simulink model "Hardmon_CAN"  (R2023b)
settings: Solver=VariableStepAuto  StartTime=0.0  StopTime=10.0  RelTol=1e-3
settings Model: Creator=heyka  LastModifiedBy=heyka

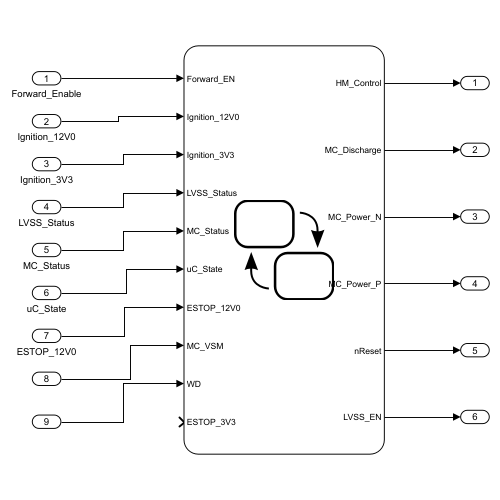
[thumbnail: Simulink's stored preview of the top-level diagram]
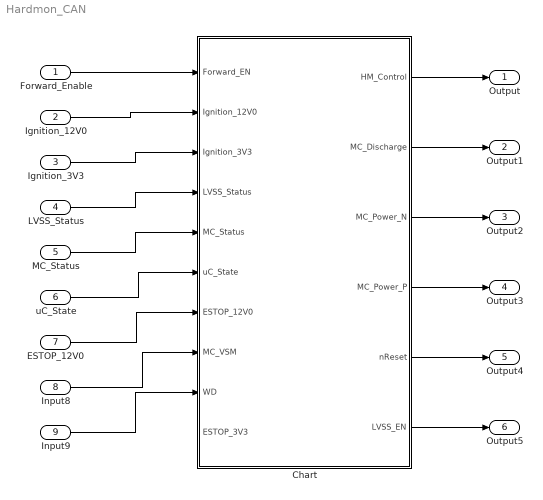
== system Hardmon_CAN ==
  Forward_Enable : Inport
  Ignition_12V0 : Inport  Port=2
  Ignition_3V3 : Inport  Port=3
  LVSS_Status : Inport  Port=4
  MC_Status : Inport  Port=5
  uC_State : Inport  Port=6
  ESTOP_12V0 : Inport  Port=7
  Input8 : Inport  Port=8
  Input9 : Inport  Port=9
  Chart : Stateflow chart  TreatAsAtomicUnit=on
  Output : Outport
  Output1 : Outport  Port=2
  Output2 : Outport  Port=3
  Output3 : Outport  Port=4
  Output4 : Outport  Port=5
  Output5 : Outport  Port=6
  wires:
  Input8/1 -> Chart/8(MC_VSM)
  uC_State/1 -> Chart/6(uC_State)
  Forward_Enable/1 -> Chart/1(Forward_EN)
  LVSS_Status/1 -> Chart/4(LVSS_Status)
  Chart/5(nReset) -> Output4/1
  Ignition_12V0/1 -> Chart/2(Ignition_12V0)
  Ignition_3V3/1 -> Chart/3(Ignition_3V3)
  ESTOP_12V0/1 -> Chart/7(ESTOP_12V0)
  MC_Status/1 -> Chart/5(MC_Status)
  Input9/1 -> Chart/9(WD)
  Chart/1(HM_Control) -> Output/1
  Chart/2(MC_Discharge) -> Output1/1
  Chart/3(MC_Power_N) -> Output2/1
  Chart/4(MC_Power_P) -> Output3/1
  Chart/6(LVSS_EN) -> Output5/1

== stateflow chart Hardmon_CAN/Chart ==
  state Normal_Operation
    state ESTOP_Checking [parallel]
      settings: executionOrder=1
      state count
        entry:
        ESTOP_Counter = ESTOP_Counter + 1;
      state ESTOP_Inactive
        entry:
        Fault = 0;
        ESTOP_Counter = 0;
        HM_Control = 0;
        LVSS_EN = 1;
      (default) -> ESTOP_Inactive
      ESTOP_Inactive -> Normal_Operation.ESTOP_Checking.count : [ESTOP_3V3 == 1]
      Normal_Operation.ESTOP_Checking.count -> ESTOP_Inactive [order 2] : [ESTOP_3V3 == 0 || uC_State == 7]
      Normal_Operation.ESTOP_Checking.count -> Normal_Operation.ESTOP_Checking.count [order 1] : after(0.5,sec)
    state Watchdog_Checking [parallel]
      settings: executionOrder=2
      state WD_Low
        entry:
        WD_Count = 0
        state Counting
          entry:
          WD_Count = WD_Count + 1
        Normal_Operation.Watchdog_Checking.WD_Low.Counting -> Normal_Operation.Watchdog_Checking.WD_Low.Counting : after(0.5, sec)
      state WD_High
        entry:
        WD_Count = 0;
        state Counting
          entry:
          WD_Count = WD_Count + 1
        Normal_Operation.Watchdog_Checking.WD_High.Counting -> Normal_Operation.Watchdog_Checking.WD_High.Counting : after(0.5, sec)
      (default) -> WD_Low
      WD_Low -> WD_High : [WD == 1]
      WD_High -> WD_Low : [WD == 0]
    state Invalid_State_Checking [parallel]
      settings: executionOrder=3
      state count
        entry:
        Invalid_State_Counter = Invalid_State_Counter + 1;
      state Invalid_State_Inactive
        entry:
        Fault = 0;
        Invalid_State_Counter = 0;
        HM_Control = 0;
        LVSS_EN = 1;
      (default) -> Normal_Operation.Invalid_State_Checking.Invalid_State_Inactive
      Normal_Operation.Invalid_State_Checking.Invalid_State_Inactive -> Normal_Operation.Invalid_State_Checking.count : [(Forward_EN ~= 1 || Ignition_3V3 ~= 1) && uC_State == 3]
      Normal_Operation.Invalid_State_Checking.count -> Normal_Operation.Invalid_State_Checking.Invalid_State_Inactive [order 2] : [~((Forward_EN ~= 1 || Ignition_3V3 ~= 1) && uC_State == 3)]
      Normal_Operation.Invalid_State_Checking.count -> Normal_Operation.Invalid_State_Checking.count [order 1] : after(0.5,sec)
    state Ignition_Level_Checking [parallel]
      settings: executionOrder=4
      state count
        entry:
        Ignition_State_Counter = Invalid_State_Counter + 1;
      state Ignition_State_Inactive
        entry:
        Fault = 0;
        Ignition_State_Counter = 0;
        HM_Control = 0;
        LVSS_EN = 1;
      (default) -> Ignition_State_Inactive
      Ignition_State_Inactive -> Normal_Operation.Ignition_Level_Checking.count : [Ignition_3V3 ~= Ignition_12V0]
      Normal_Operation.Ignition_Level_Checking.count -> Ignition_State_Inactive [order 2] : [Ignition_3V3 == Ignition_12V0]
      Normal_Operation.Ignition_Level_Checking.count -> Normal_Operation.Ignition_Level_Checking.count [order 1] : after(0.5,sec)
    state ESTOP_Level_Checking [parallel]
      settings: executionOrder=5
      state count
        entry:
        ESTOP_State_Counter = ESTOP_State_Counter + 1;
      state ESTOP_State_Inactive
        entry:
        Fault = 0;
        ESTOP_State_Counter = 0;
        HM_Control = 0;
        LVSS_EN = 1;
      (default) -> ESTOP_State_Inactive
      ESTOP_State_Inactive -> Normal_Operation.ESTOP_Level_Checking.count : [ESTOP_3V3 ~= ESTOP_12V0]
      Normal_Operation.ESTOP_Level_Checking.count -> ESTOP_State_Inactive [order 2] : [ESTOP_3V3 == ESTOP_12V0]
      Normal_Operation.ESTOP_Level_Checking.count -> Normal_Operation.ESTOP_Level_Checking.count [order 1] : after(0.5,sec)
    state LVSS_Checking [parallel]
      settings: executionOrder=6
      state count
        entry:
        LVSS_Counter = LVSS_Counter + 1;
      state Invalid_State_Inactive
        entry:
        Fault = 0;
        LVSS_Counter = 0;
        HM_Control = 0;
      (default) -> Normal_Operation.LVSS_Checking.Invalid_State_Inactive
      Normal_Operation.LVSS_Checking.Invalid_State_Inactive -> Normal_Operation.LVSS_Checking.count : [LVSS_Status ~= LVSS_EN]
      Normal_Operation.LVSS_Checking.count -> Normal_Operation.LVSS_Checking.Invalid_State_Inactive [order 2] : [LVSS_Status == LVSS_EN]
      Normal_Operation.LVSS_Checking.count -> Normal_Operation.LVSS_Checking.count [order 1] : after(0.5,sec)
  state MC_DISCHARGE
    entry:
    nReset = 0;
    HM_Control = 1;
    MC_Discharge = 1;
  state MC_POWERDOWN
    entry:
    MC_Discharge = 0;
    MC_Power_P = 0;
    MC_Power_N = 1;
    exit:
    MC_Power_P = 0;
    MC_Power_N = 0;
  state LVSS_Powerdown
    entry:
    LVSS_EN = 0;
  state Enter_Fault
    entry:
    nReset = 1;
    Fault = 1;
    exit:
    HM_Control = 0;
  (default) -> Normal_Operation
  Normal_Operation -> MC_DISCHARGE : [ESTOP_Counter >= 4 || WD_Count >= 4 || Invalid_State_Counter >= 4 || Ignition_State_Counter >= 4 || LVSS_Counter >=4]
  MC_DISCHARGE -> MC_POWERDOWN : [MC_VSM == 4]
  MC_POWERDOWN -> LVSS_Powerdown : [MC_Status == 0]
  LVSS_Powerdown -> Enter_Fault : [LVSS_Status == 0]
  Enter_Fault -> Normal_Operation : [uC_State == 6]
  data: WD_Count local; Forward_EN input; Ignition_12V0 input; Ignition_3V3 input; LVSS_Status input; MC_Status input; uC_State input; Fault local; HM_Control output; MC_Discharge output; MC_Power_N output; MC_Power_P output; nReset output; ESTOP_State_Counter local; Ignition_State_Counter local; Invalid_State_Counter local; LVSS_Counter local; LVSS_EN output; ESTOP_12V0 input; MC_VSM input; WD input; ESTOP_Counter local; ESTOP_3V3 input =0
